simulink model "model"  (R2019b)
settings: Solver=VariableStepAuto  StartTime=0.0  StopTime=10.0  RelTol=1e-3
values from neighbouring files (symbols this model uses):
  DH = zeros(n,4)    [create_rob.m]    (also in createrobot.m = [DH; [theta_vec(i) d_vec(i) a_vec(i) alpha_vec(i)]])
  qtype = text(2:1+n)'    [create_rob.m]    (also in createrobot.m = [0, 0, 0]; normalize.m = evalin('base','qtype'))
settings Model: Creator=lucas  LastModifiedBy=lucas
settings DebuggingCC: UnderSpecifiedDimensionMsg=error

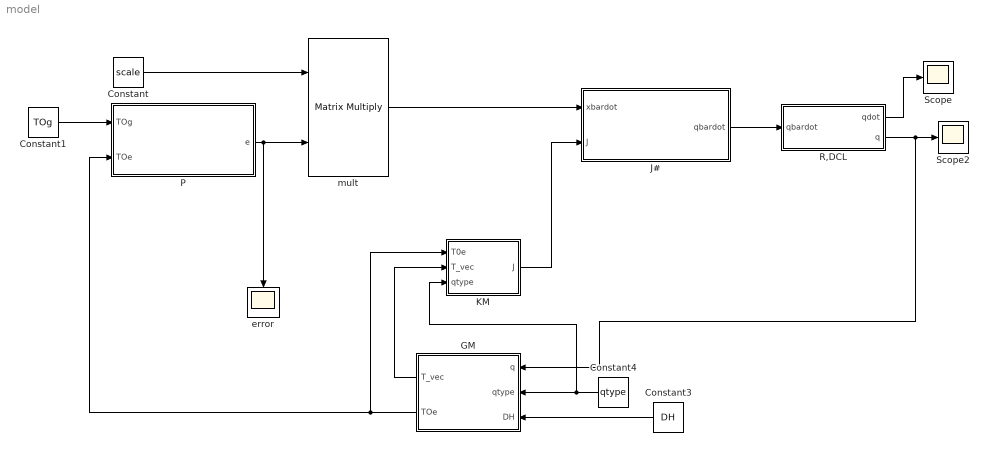
== system model ==
  Constant : Constant  Value=scale  mask{scale=55*eye(6)}
  Constant1 : Constant  Value=TOg  mask{TOg=[eye(3), [0; 0; 0]; zeros(1,4)]}
  Constant3 : Constant  Value=DH
  Constant4 : Constant  Value=qtype
  GM : Subsystem
  J# : MATLAB Function  TreatAsAtomicUnit=on
  KM : MATLAB Function  TreatAsAtomicUnit=on
  P : MATLAB Function  TreatAsAtomicUnit=on
  R,DCL : Subsystem
  Scope : Scope
  Scope2 : Scope
  error : Scope
  mult : Product  Multiplication=Matrix(*)
  wires:
  Constant/1 -> mult/1
  Constant1/1 -> P/1(TOg)
  R,DCL/1(qdot) -> Scope/1
  R,DCL/2(q) -> GM/1(q), Scope2/1
  P/1(e) -> mult/2, error/1
  J#/1(qbardot) -> R,DCL/1(qbardot)
  KM/1(J) -> J#/2(J)
  mult/1 -> J#/1(xbardot)
  Constant4/1 -> KM/3(qtype), GM/2(qtype)
  Constant3/1 -> GM/3(DH)
  GM/1(T_vec) -> KM/2(T_vec)
  GM/2(TOe) -> KM/1(T0e), P/2(TOe)

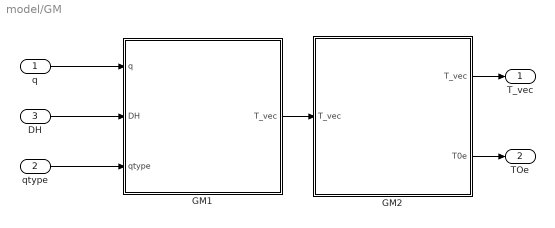
== system model/GM ==
  q : Inport
  qtype : Inport  Port=2
  DH : Inport  Port=3
  GM1 : MATLAB Function  TreatAsAtomicUnit=on
  GM2 : MATLAB Function  TreatAsAtomicUnit=on
  T_vec : Outport
  TOe : Outport  Port=2
  wires:
  DH/1 -> GM1/2(DH)
  q/1 -> GM1/1(q)
  qtype/1 -> GM1/3(qtype)
  GM1/1(T_vec) -> GM2/1("T_vec ")
  GM2/2(T0e) -> TOe/1
  GM2/1(T_vec) -> T_vec/1

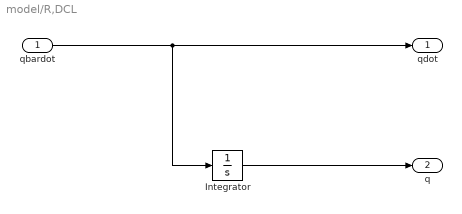
== system model/R,DCL ==
  qbardot : Inport
  Integrator : Integrator
  qdot : Outport
  q : Outport  Port=2
  wires:
  qbardot/1 -> Integrator/1, qdot/1
  Integrator/1 -> q/1

== matlab function model/J# ==
  data: xbardot input; qbardot output; J input
function qbardot = fcn(xbardot,J)
    
    [U,Sigma,V] = svd(J);
    Sigmasharp = pinv(Sigma);
   
%     l = rank(Sigmasharp);
%     thr = 0.01;
%     
%     for i = 1 : l
%        singval = Sigma(i,i);
%        if singval > thr
%            psquare = 0;
%        else
%            psquare = 300;
%            'reg'
%        end
%        Sigmasharp(i,i) = singval / (singval^2 + psquare);
%     end
    
    JSharp = V * Sigmasharp * U.';
    qbardot = JSharp * xbardot;

end

== matlab function model/P ==
  data: TOg input; e output; TOe input
function e = fcn(TOg,TOe)
    %a
    % R = Rab
    %b
    
    e = zeros(6,1);
    
    ROg = TOg(1:3,1:3); % extract the rotation part
    ROe = TOe(1:3,1:3); % extract the rotation part
    Reg = ROe.' * ROg;
    
    % delta = costheta, rho = vtheta
    delta = (trace(Reg) - 1)/2;
    
    eie = [1; 0; 0];
    eje = [0; 1; 0];
    eke = [0; 0; 1];
    eig = Reg(1:3,1);
    ejg = Reg(1:3,2);
    ekg = Reg(1:3,3);
    
    % axb means a ^ b
    ixi = cross(eie, eig);
    jxj = cross(eje, ejg);
    kxk = cross(eke, ekg);
    sigma = 0.5 * (ixi + jxj + kxk);
    
    if (delta == 1) 
       v = [0; 0; 0];
       theta = 0;
    elseif (delta == -1)
        sumijk = eie + eje + eke + eig + ejg + ekg;
        v = (sumijk) / norm(sumijk);
        theta = pi;
    else
        v = sigma / norm(sigma);
        theta = atan2(norm(sigma),delta);
    end
    
    e(1:3) = v*theta;
    e(4:6) = TOg(1:3,4) - TOe(1:3,4);
    
    
end

== matlab function model/KM ==
  data: T0e input; J output size=[6 n]; T_vec input; qtype input
function J = fcn(T0e, T_vec, qtype)

    Tsize = size(T_vec);
    n = Tsize(3);
    
    % Initialize Jacobian
    J = zeros(6,n);
    
    OOe = T0e(1:3,4);
    
    for i = 1 : n
        T0toi = eye(4,4); % T matrix from 0 to i
        for l = 1 : i
            % T0toi = prod of previous T matrices
            T0toi = T0toi * T_vec(:,:,l);
        end
        
        % ki projected on 0
        ki = T0toi(1:3,3);
        
        % distance from O to O1
        OOi = T0toi(1:3,4);
        
        if qtype(i) == 0 % rot joint
            rei = OOe - OOi; % ray vector from i to e
            J(:, i) = [ki; cross(ki, rei)];
        else % prismatic joint
            J(:, i) = [zeros(3,1); ki]; 
        end
    end 
end

== matlab function model/GM/GM1 ==
  data: q input; T_vec output size=[4 4 n]; DH input; qtype input
function T_vec = gm1 (q, DH, qtype)

    % DH = each row has, in order, theta, d, a, alpha
    qsize = size(q);
    n = qsize(1);
    T_vec = zeros(4,4,n);
    
    for i = 1:n
        T_bar = r2t(rotz(DH(i,1))) * transl(0, 0, DH(i,2)) ...
            * transl(DH(i,3), 0, 0) * r2t(rotx(DH(i,4)));
        
        % qtype(i) is 0 if rot, 1 if transl
        if (qtype(i) == 0)
            % rotational joint
            T_q = r2t(rotz(q(i)));
        elseif (qtype(i) == 1)
            % translational joint
            T_q = transl(0, 0, q(i));
        else
            error('joint not recognized');
        end
        
        % T_vec{1, i} is the transformation matrix from frame i - 1 to
        % frame i
        T_vec(:,:,i) = T_bar * T_q;
    end
end

== matlab function model/GM/GM2 ==
  data: T_vec output; T_vec input; T0e output
function [T_vec, T0e] = gm2 (T_vec)
    
    Tsize = size(T_vec);
    n = Tsize(3);
    T0e = eye(4,4);
    
    for i = 1 : n
        T0e = T0e * T_vec(:,:,i);
    end
    
end
